simulink model "TST_EISGov_TrqLosEst"  (R2016b)
settings: Solver=FixedStepDiscrete  StartTime=0.0  StopTime=0.02  FixedStep=sampleTime  RelTol=1e-3
values from neighbouring files (symbols this model uses):
  testCase = 1    [initTST_EISGov_TrqLosEst_001.m]    (also in initTST_EISGov_TrqLosEst_002.m = 2; initTST_EISGov_TrqLosEst_003.m = 3; initTST_EISGov_TrqLosEst_004.m = 4)
libraries: simulink x9, UnitTest_Lib x4
settings Model: Creator=zhengjinyan  LastModifiedBy=zhengjinyan
settings DebuggingCC: SignalRangeChecking=error

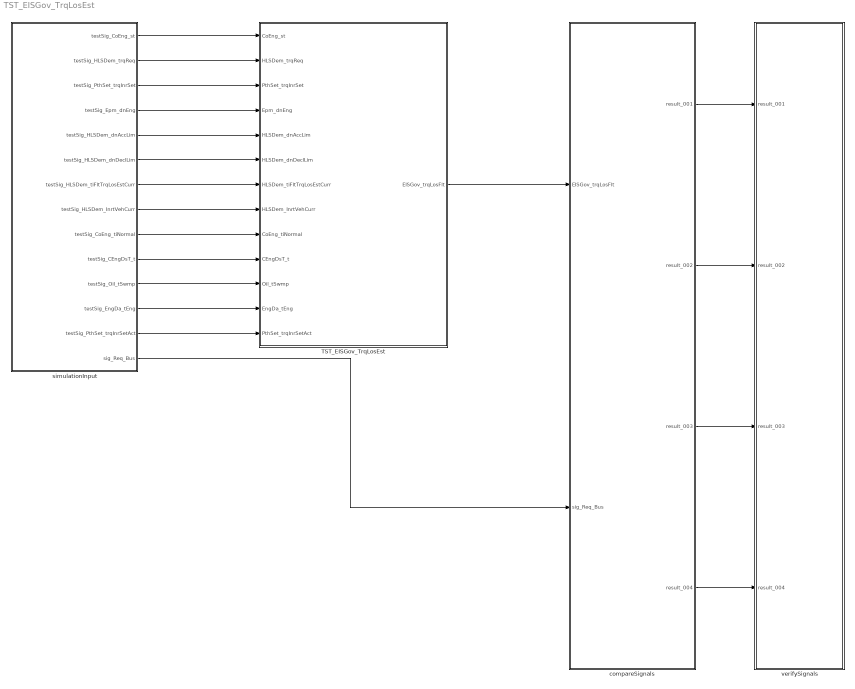
== system TST_EISGov_TrqLosEst ==
  TST_EISGov_TrqLosEst : Subsystem
  compareSignals : Subsystem
  simulationInput : Subsystem
  verifySignals : Subsystem
  wires:
  simulationInput/1(testSig_CoEng_st) -> TST_EISGov_TrqLosEst/1(CoEng_st)
  simulationInput/2(testSig_HLSDem_trqReq) -> TST_EISGov_TrqLosEst/2(HLSDem_trqReq)
  simulationInput/3(testSig_PthSet_trqInrSet) -> TST_EISGov_TrqLosEst/3(PthSet_trqInrSet)
  simulationInput/4(testSig_Epm_dnEng) -> TST_EISGov_TrqLosEst/4(Epm_dnEng)
  simulationInput/5(testSig_HLSDem_dnAccLim) -> TST_EISGov_TrqLosEst/5(HLSDem_dnAccLim)
  simulationInput/6(testSig_HLSDem_dnDeclLim) -> TST_EISGov_TrqLosEst/6(HLSDem_dnDeclLim)
  simulationInput/7(testSig_HLSDem_tiFltTrqLosEstCurr) -> TST_EISGov_TrqLosEst/7(HLSDem_tiFltTrqLosEstCurr)
  simulationInput/8(testSig_HLSDem_InrtVehCurr) -> TST_EISGov_TrqLosEst/8(HLSDem_InrtVehCurr)
  simulationInput/9(testSig_CoEng_tiNormal) -> TST_EISGov_TrqLosEst/9(CoEng_tiNormal)
  simulationInput/10(testSig_CEngDsT_t) -> TST_EISGov_TrqLosEst/10(CEngDsT_t)
  simulationInput/11(testSig_Oil_tSwmp) -> TST_EISGov_TrqLosEst/11(Oil_tSwmp)
  simulationInput/12(testSig_EngDa_tEng) -> TST_EISGov_TrqLosEst/12(EngDa_tEng)
  simulationInput/13(testSig_PthSet_trqInrSetAct) -> TST_EISGov_TrqLosEst/13(PthSet_trqInrSetAct)
  TST_EISGov_TrqLosEst/1(EISGov_trqLosFlt) -> compareSignals/1(EISGov_trqLosFlt)
  simulationInput/14(sig_Req_Bus) -> compareSignals/2(sig_Req_Bus)
  compareSignals/1(result_001) -> verifySignals/1(result_001)
  compareSignals/2(result_002) -> verifySignals/2(result_002)
  compareSignals/3(result_003) -> verifySignals/3(result_003)
  compareSignals/4(result_004) -> verifySignals/4(result_004)

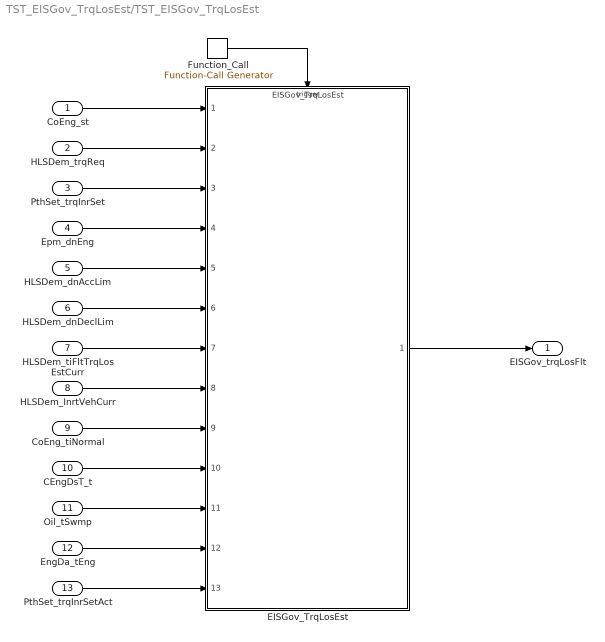
== system TST_EISGov_TrqLosEst/TST_EISGov_TrqLosEst ==
  CoEng_st : Inport
  HLSDem_trqReq : Inport  Port=2
  PthSet_trqInrSet : Inport  Port=3
  Epm_dnEng : Inport  Port=4
  HLSDem_dnAccLim : Inport  Port=5
  HLSDem_dnDeclLim : Inport  Port=6
  HLSDem_tiFltTrqLosEstCurr : Inport  Port=7
  HLSDem_InrtVehCurr : Inport  Port=8
  CoEng_tiNormal : Inport  Port=9
  CEngDsT_t : Inport  Port=10
  Oil_tSwmp : Inport  Port=11
  EngDa_tEng : Inport  Port=12
  PthSet_trqInrSetAct : Inport  Port=13
  EISGov_TrqLosEst : ModelReference  ModelNameDialog=EISGov_TrqLosEst  SimulationMode=Normal  ModelReferenceVersion=1.93  TriggerPortName=function  TriggerPortTriggerType=function-call  TriggerPortStatesWhenEnabling=held
  Function_Call : simulink/Ports & Subsystems/Function-Call Generator  sample_time=sampleTime  numberOfIterations=1
  EISGov_trqLosFlt : Outport
  wires:
  Function_Call/1 -> EISGov_TrqLosEst/Trigger
  CoEng_st/1 -> EISGov_TrqLosEst/1
  HLSDem_trqReq/1 -> EISGov_TrqLosEst/2
  PthSet_trqInrSet/1 -> EISGov_TrqLosEst/3
  Epm_dnEng/1 -> EISGov_TrqLosEst/4
  HLSDem_dnAccLim/1 -> EISGov_TrqLosEst/5
  HLSDem_dnDeclLim/1 -> EISGov_TrqLosEst/6
  HLSDem_tiFltTrqLosEstCurr/1 -> EISGov_TrqLosEst/7
  HLSDem_InrtVehCurr/1 -> EISGov_TrqLosEst/8
  CoEng_tiNormal/1 -> EISGov_TrqLosEst/9
  CEngDsT_t/1 -> EISGov_TrqLosEst/10
  Oil_tSwmp/1 -> EISGov_TrqLosEst/11
  EngDa_tEng/1 -> EISGov_TrqLosEst/12
  PthSet_trqInrSetAct/1 -> EISGov_TrqLosEst/13
  EISGov_TrqLosEst/1 -> EISGov_trqLosFlt/1

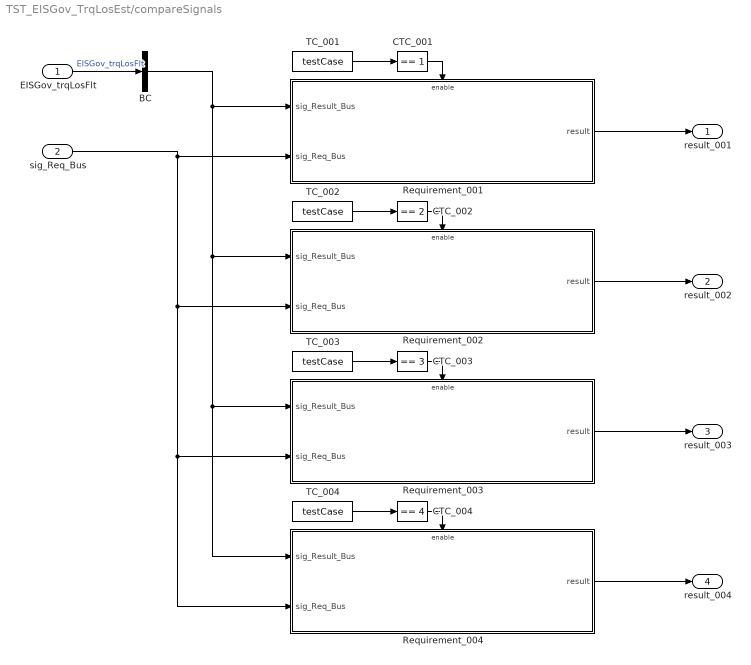
== system TST_EISGov_TrqLosEst/compareSignals ==
  EISGov_trqLosFlt : Inport
  sig_Req_Bus : Inport  Port=2
  BC : BusCreator  Inputs=1
  CTC_001 : simulink/Logic and Bit Operations/Compare To Constant  relop===  const=1  OutDataTypeStr=boolean
  CTC_002 : simulink/Logic and Bit Operations/Compare To Constant  relop===  const=2  OutDataTypeStr=boolean
  CTC_003 : simulink/Logic and Bit Operations/Compare To Constant  relop===  const=3  OutDataTypeStr=boolean
  CTC_004 : simulink/Logic and Bit Operations/Compare To Constant  relop===  const=4  OutDataTypeStr=boolean
  Requirement_001 : Subsystem
  Requirement_002 : Subsystem
  Requirement_003 : Subsystem
  Requirement_004 : Subsystem
  TC_001 : Constant  Value=testCase
  TC_002 : Constant  Value=testCase
  TC_003 : Constant  Value=testCase
  TC_004 : Constant  Value=testCase
  result_001 : Outport
  result_002 : Outport  Port=2
  result_003 : Outport  Port=3
  result_004 : Outport  Port=4
  wires:
  EISGov_trqLosFlt/1 -> BC/1  "EISGov_trqLosFlt"
  TC_001/1 -> CTC_001/1
  CTC_001/1 -> Requirement_001/Enable
  sig_Req_Bus/1 -> Requirement_003/2(sig_Req_Bus), Requirement_004/2(sig_Req_Bus), Requirement_002/2(sig_Req_Bus), Requirement_001/2(sig_Req_Bus)
  BC/1 -> Requirement_003/1(sig_Result_Bus), Requirement_004/1(sig_Result_Bus), Requirement_002/1(sig_Result_Bus), Requirement_001/1(sig_Result_Bus)
  Requirement_001/1(result) -> result_001/1
  TC_002/1 -> CTC_002/1
  CTC_002/1 -> Requirement_002/Enable
  Requirement_002/1(result) -> result_002/1
  TC_003/1 -> CTC_003/1
  CTC_003/1 -> Requirement_003/Enable
  Requirement_003/1(result) -> result_003/1
  TC_004/1 -> CTC_004/1
  CTC_004/1 -> Requirement_004/Enable
  Requirement_004/1(result) -> result_004/1

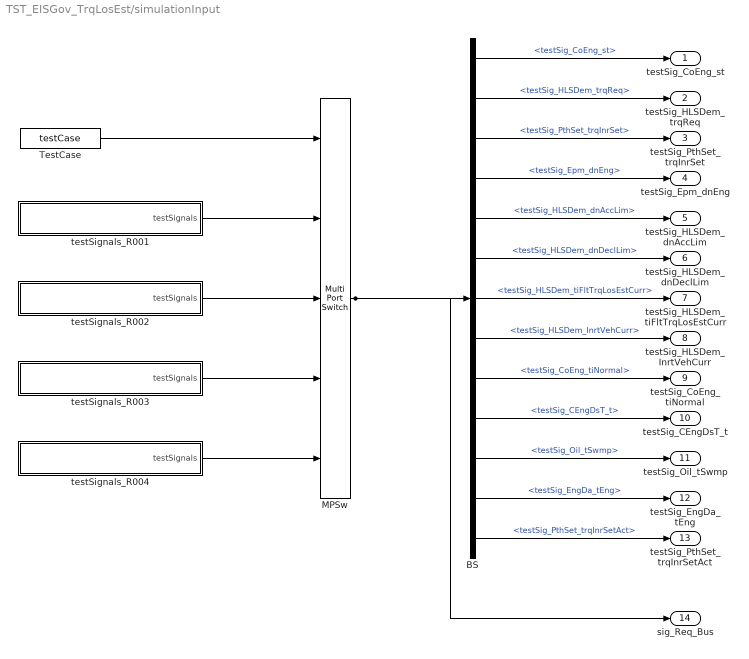
== system TST_EISGov_TrqLosEst/simulationInput ==
  BS : BusSelector  OutputSignals=testSig_CoEng_st,testSig_HLSDem_trqReq,testSig_PthSet_trqInrSet,testSig_Epm_dnEng,testSig_HLSDem_dnAccLim,testSig_HLSDem_dnDeclLim,testSig_HLSDem_tiFltTrqLosEstCurr,testSig_HLSDem_InrtVehCurr,testSig_CoEng_tiNormal,testSig_CEngDsT_t,testSig_Oil_tSwmp,testSig_EngDa_tEng,testSig_PthSet_trqInrSetAct
  MPSw : MultiPortSwitch  Inputs=4  SaturateOnIntegerOverflow=on  InputSameDT=on
  TestCase : Constant  Value=testCase
  testSignals_R001 : Subsystem
  testSignals_R002 : Subsystem
  testSignals_R003 : Subsystem
  testSignals_R004 : Subsystem
  testSig_CoEng_st : Outport
  testSig_HLSDem_trqReq : Outport  Port=2
  testSig_PthSet_trqInrSet : Outport  Port=3
  testSig_Epm_dnEng : Outport  Port=4
  testSig_HLSDem_dnAccLim : Outport  Port=5
  testSig_HLSDem_dnDeclLim : Outport  Port=6
  testSig_HLSDem_tiFltTrqLosEstCurr : Outport  Port=7
  testSig_HLSDem_InrtVehCurr : Outport  Port=8
  testSig_CoEng_tiNormal : Outport  Port=9
  testSig_CEngDsT_t : Outport  Port=10
  testSig_Oil_tSwmp : Outport  Port=11
  testSig_EngDa_tEng : Outport  Port=12
  testSig_PthSet_trqInrSetAct : Outport  Port=13
  sig_Req_Bus : Outport  Port=14
  wires:
  BS/1 -> testSig_CoEng_st/1  "<testSig_CoEng_st>"
  BS/2 -> testSig_HLSDem_trqReq/1  "<testSig_HLSDem_trqReq>"
  BS/3 -> testSig_PthSet_trqInrSet/1  "<testSig_PthSet_trqInrSet>"
  BS/4 -> testSig_Epm_dnEng/1  "<testSig_Epm_dnEng>"
  BS/5 -> testSig_HLSDem_dnAccLim/1  "<testSig_HLSDem_dnAccLim>"
  BS/6 -> testSig_HLSDem_dnDeclLim/1  "<testSig_HLSDem_dnDeclLim>"
  BS/7 -> testSig_HLSDem_tiFltTrqLosEstCurr/1  "<testSig_HLSDem_tiFltTrqLosEstCurr>"
  BS/8 -> testSig_HLSDem_InrtVehCurr/1  "<testSig_HLSDem_InrtVehCurr>"
  BS/9 -> testSig_CoEng_tiNormal/1  "<testSig_CoEng_tiNormal>"
  BS/10 -> testSig_CEngDsT_t/1  "<testSig_CEngDsT_t>"
  BS/11 -> testSig_Oil_tSwmp/1  "<testSig_Oil_tSwmp>"
  BS/12 -> testSig_EngDa_tEng/1  "<testSig_EngDa_tEng>"
  BS/13 -> testSig_PthSet_trqInrSetAct/1  "<testSig_PthSet_trqInrSetAct>"
  MPSw/1 -> BS/1, sig_Req_Bus/1
  TestCase/1 -> MPSw/1
  testSignals_R001/1(testSignals) -> MPSw/2
  testSignals_R002/1(testSignals) -> MPSw/3
  testSignals_R003/1(testSignals) -> MPSw/4
  testSignals_R004/1(testSignals) -> MPSw/5

== system TST_EISGov_TrqLosEst/verifySignals ==
  result_001 : Inport
  result_002 : Inport  Port=2
  result_003 : Inport  Port=3
  result_004 : Inport  Port=4
  Assertion_001 : Assertion  Enabled=off
  Assertion_002 : Assertion
  Assertion_003 : Assertion  Enabled=off
  Assertion_004 : Assertion  Enabled=off
  wires:
  result_001/1 -> Assertion_001/1
  result_002/1 -> Assertion_002/1
  result_003/1 -> Assertion_003/1
  result_004/1 -> Assertion_004/1

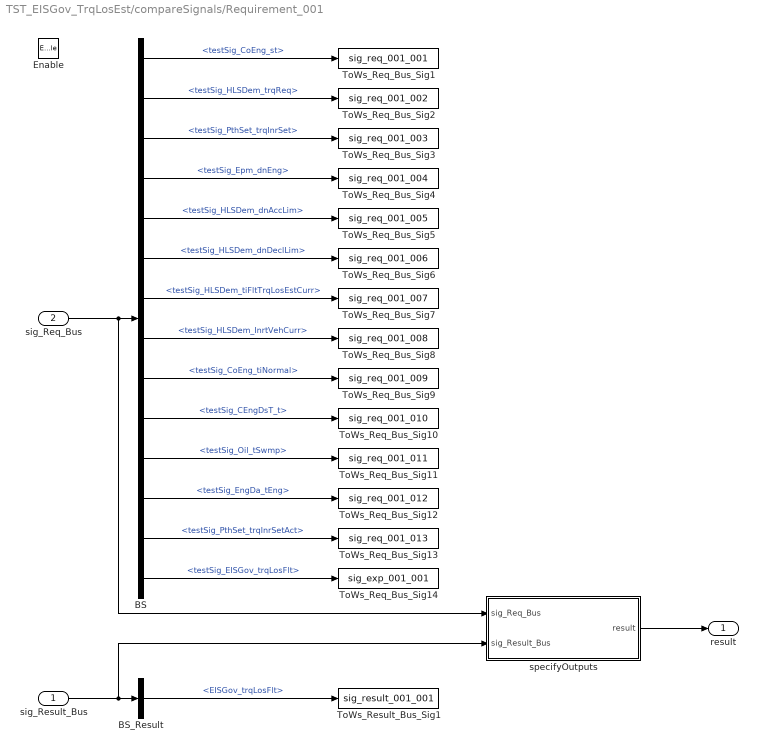
== system TST_EISGov_TrqLosEst/compareSignals/Requirement_001 ==
  sig_Result_Bus : Inport
  sig_Req_Bus : Inport  Port=2
  Enable : EnablePort
  BS : BusSelector  OutputSignals=testSig_CoEng_st,testSig_HLSDem_trqReq,testSig_PthSet_trqInrSet,testSig_Epm_dnEng,testSig_HLSDem_dnAccLim,testSig_HLSDem_dnDeclLim,testSig_HLSDem_tiFltTrqLosEstCurr,testSig_HLSDem_InrtVehCurr,testSig_CoEng_tiNormal,testSig_CEngDsT_t,testSig_Oil_tSwmp,testSig_EngDa_tEng,testSig_PthSet_trqInrSetAct,testSig_EISGov_trqLosFlt
  BS_Result : BusSelector  OutputSignals=EISGov_trqLosFlt
  ToWs_Req_Bus_Sig1 : ToWorkspace  VariableName=sig_req_001_001  SaveFormat=Structure With Time
  ToWs_Req_Bus_Sig10 : ToWorkspace  VariableName=sig_req_001_010  SaveFormat=Structure With Time
  ToWs_Req_Bus_Sig11 : ToWorkspace  VariableName=sig_req_001_011  SaveFormat=Structure With Time
  ToWs_Req_Bus_Sig12 : ToWorkspace  VariableName=sig_req_001_012  SaveFormat=Structure With Time
  ToWs_Req_Bus_Sig13 : ToWorkspace  VariableName=sig_req_001_013  SaveFormat=Structure With Time
  ToWs_Req_Bus_Sig14 : ToWorkspace  VariableName=sig_exp_001_001  SaveFormat=Structure With Time
  ToWs_Req_Bus_Sig2 : ToWorkspace  VariableName=sig_req_001_002  SaveFormat=Structure With Time
  ToWs_Req_Bus_Sig3 : ToWorkspace  VariableName=sig_req_001_003  SaveFormat=Structure With Time
  ToWs_Req_Bus_Sig4 : ToWorkspace  VariableName=sig_req_001_004  SaveFormat=Structure With Time
  ToWs_Req_Bus_Sig5 : ToWorkspace  VariableName=sig_req_001_005  SaveFormat=Structure With Time
  ToWs_Req_Bus_Sig6 : ToWorkspace  VariableName=sig_req_001_006  SaveFormat=Structure With Time
  ToWs_Req_Bus_Sig7 : ToWorkspace  VariableName=sig_req_001_007  SaveFormat=Structure With Time
  ToWs_Req_Bus_Sig8 : ToWorkspace  VariableName=sig_req_001_008  SaveFormat=Structure With Time
  ToWs_Req_Bus_Sig9 : ToWorkspace  VariableName=sig_req_001_009  SaveFormat=Structure With Time
  ToWs_Result_Bus_Sig1 : ToWorkspace  VariableName=sig_result_001_001  SaveFormat=Structure With Time
  specifyOutputs : Subsystem
  result : Outport
  wires:
  sig_Req_Bus/1 -> BS/1, specifyOutputs/1(sig_Req_Bus)
  BS/1 -> ToWs_Req_Bus_Sig1/1  "<testSig_CoEng_st>"
  BS/2 -> ToWs_Req_Bus_Sig2/1  "<testSig_HLSDem_trqReq>"
  BS/3 -> ToWs_Req_Bus_Sig3/1  "<testSig_PthSet_trqInrSet>"
  BS/4 -> ToWs_Req_Bus_Sig4/1  "<testSig_Epm_dnEng>"
  BS/5 -> ToWs_Req_Bus_Sig5/1  "<testSig_HLSDem_dnAccLim>"
  BS/6 -> ToWs_Req_Bus_Sig6/1  "<testSig_HLSDem_dnDeclLim>"
  BS/7 -> ToWs_Req_Bus_Sig7/1  "<testSig_HLSDem_tiFltTrqLosEstCurr>"
  BS/8 -> ToWs_Req_Bus_Sig8/1  "<testSig_HLSDem_InrtVehCurr>"
  BS/9 -> ToWs_Req_Bus_Sig9/1  "<testSig_CoEng_tiNormal>"
  BS/10 -> ToWs_Req_Bus_Sig10/1  "<testSig_CEngDsT_t>"
  BS/11 -> ToWs_Req_Bus_Sig11/1  "<testSig_Oil_tSwmp>"
  BS/12 -> ToWs_Req_Bus_Sig12/1  "<testSig_EngDa_tEng>"
  BS/13 -> ToWs_Req_Bus_Sig13/1  "<testSig_PthSet_trqInrSetAct>"
  BS/14 -> ToWs_Req_Bus_Sig14/1  "<testSig_EISGov_trqLosFlt>"
  sig_Result_Bus/1 -> BS_Result/1, specifyOutputs/2(sig_Result_Bus)
  BS_Result/1 -> ToWs_Result_Bus_Sig1/1  "<EISGov_trqLosFlt>"
  specifyOutputs/1(result) -> result/1

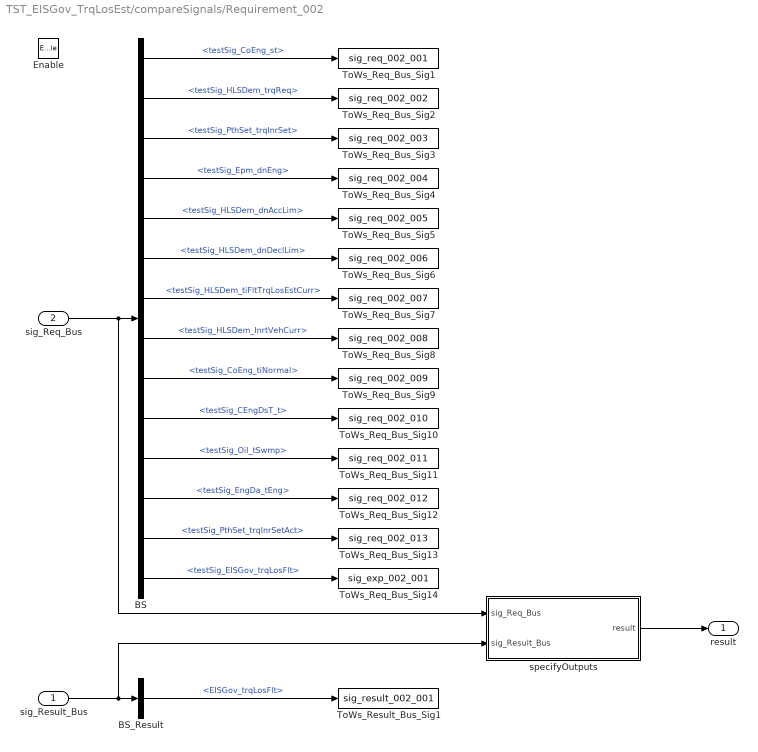
== system TST_EISGov_TrqLosEst/compareSignals/Requirement_002 ==
  sig_Result_Bus : Inport
  sig_Req_Bus : Inport  Port=2
  Enable : EnablePort
  BS : BusSelector  OutputSignals=testSig_CoEng_st,testSig_HLSDem_trqReq,testSig_PthSet_trqInrSet,testSig_Epm_dnEng,testSig_HLSDem_dnAccLim,testSig_HLSDem_dnDeclLim,testSig_HLSDem_tiFltTrqLosEstCurr,testSig_HLSDem_InrtVehCurr,testSig_CoEng_tiNormal,testSig_CEngDsT_t,testSig_Oil_tSwmp,testSig_EngDa_tEng,testSig_PthSet_trqInrSetAct,testSig_EISGov_trqLosFlt
  BS_Result : BusSelector  OutputSignals=EISGov_trqLosFlt
  ToWs_Req_Bus_Sig1 : ToWorkspace  VariableName=sig_req_002_001  SaveFormat=Structure With Time
  ToWs_Req_Bus_Sig10 : ToWorkspace  VariableName=sig_req_002_010  SaveFormat=Structure With Time
  ToWs_Req_Bus_Sig11 : ToWorkspace  VariableName=sig_req_002_011  SaveFormat=Structure With Time
  ToWs_Req_Bus_Sig12 : ToWorkspace  VariableName=sig_req_002_012  SaveFormat=Structure With Time
  ToWs_Req_Bus_Sig13 : ToWorkspace  VariableName=sig_req_002_013  SaveFormat=Structure With Time
  ToWs_Req_Bus_Sig14 : ToWorkspace  VariableName=sig_exp_002_001  SaveFormat=Structure With Time
  ToWs_Req_Bus_Sig2 : ToWorkspace  VariableName=sig_req_002_002  SaveFormat=Structure With Time
  ToWs_Req_Bus_Sig3 : ToWorkspace  VariableName=sig_req_002_003  SaveFormat=Structure With Time
  ToWs_Req_Bus_Sig4 : ToWorkspace  VariableName=sig_req_002_004  SaveFormat=Structure With Time
  ToWs_Req_Bus_Sig5 : ToWorkspace  VariableName=sig_req_002_005  SaveFormat=Structure With Time
  ToWs_Req_Bus_Sig6 : ToWorkspace  VariableName=sig_req_002_006  SaveFormat=Structure With Time
  ToWs_Req_Bus_Sig7 : ToWorkspace  VariableName=sig_req_002_007  SaveFormat=Structure With Time
  ToWs_Req_Bus_Sig8 : ToWorkspace  VariableName=sig_req_002_008  SaveFormat=Structure With Time
  ToWs_Req_Bus_Sig9 : ToWorkspace  VariableName=sig_req_002_009  SaveFormat=Structure With Time
  ToWs_Result_Bus_Sig1 : ToWorkspace  VariableName=sig_result_002_001  SaveFormat=Structure With Time
  specifyOutputs : Subsystem
  result : Outport
  wires:
  sig_Req_Bus/1 -> BS/1, specifyOutputs/1(sig_Req_Bus)
  BS/1 -> ToWs_Req_Bus_Sig1/1  "<testSig_CoEng_st>"
  BS/2 -> ToWs_Req_Bus_Sig2/1  "<testSig_HLSDem_trqReq>"
  BS/3 -> ToWs_Req_Bus_Sig3/1  "<testSig_PthSet_trqInrSet>"
  BS/4 -> ToWs_Req_Bus_Sig4/1  "<testSig_Epm_dnEng>"
  BS/5 -> ToWs_Req_Bus_Sig5/1  "<testSig_HLSDem_dnAccLim>"
  BS/6 -> ToWs_Req_Bus_Sig6/1  "<testSig_HLSDem_dnDeclLim>"
  BS/7 -> ToWs_Req_Bus_Sig7/1  "<testSig_HLSDem_tiFltTrqLosEstCurr>"
  BS/8 -> ToWs_Req_Bus_Sig8/1  "<testSig_HLSDem_InrtVehCurr>"
  BS/9 -> ToWs_Req_Bus_Sig9/1  "<testSig_CoEng_tiNormal>"
  BS/10 -> ToWs_Req_Bus_Sig10/1  "<testSig_CEngDsT_t>"
  BS/11 -> ToWs_Req_Bus_Sig11/1  "<testSig_Oil_tSwmp>"
  BS/12 -> ToWs_Req_Bus_Sig12/1  "<testSig_EngDa_tEng>"
  BS/13 -> ToWs_Req_Bus_Sig13/1  "<testSig_PthSet_trqInrSetAct>"
  BS/14 -> ToWs_Req_Bus_Sig14/1  "<testSig_EISGov_trqLosFlt>"
  sig_Result_Bus/1 -> BS_Result/1, specifyOutputs/2(sig_Result_Bus)
  BS_Result/1 -> ToWs_Result_Bus_Sig1/1  "<EISGov_trqLosFlt>"
  specifyOutputs/1(result) -> result/1

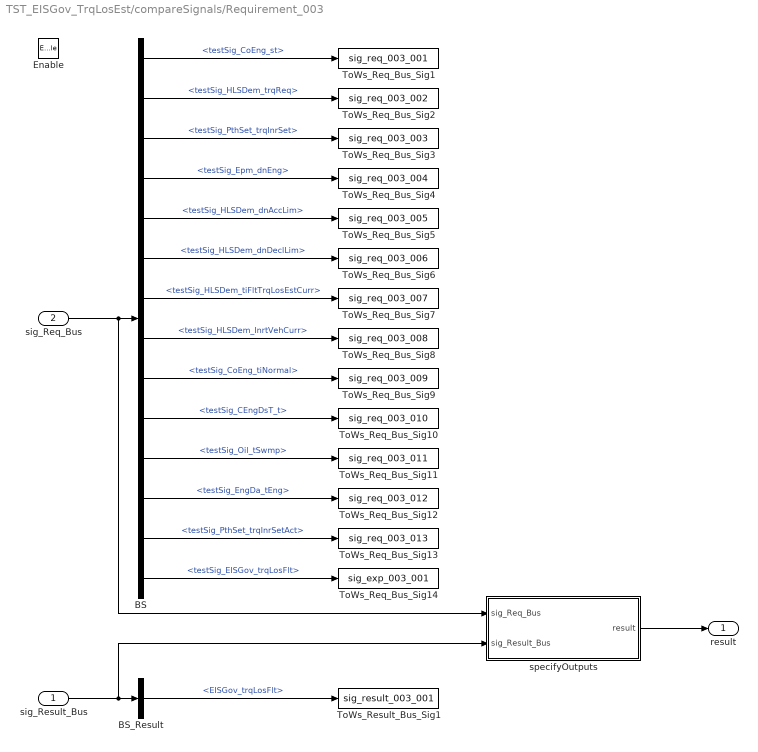
== system TST_EISGov_TrqLosEst/compareSignals/Requirement_003 ==
  sig_Result_Bus : Inport
  sig_Req_Bus : Inport  Port=2
  Enable : EnablePort
  BS : BusSelector  OutputSignals=testSig_CoEng_st,testSig_HLSDem_trqReq,testSig_PthSet_trqInrSet,testSig_Epm_dnEng,testSig_HLSDem_dnAccLim,testSig_HLSDem_dnDeclLim,testSig_HLSDem_tiFltTrqLosEstCurr,testSig_HLSDem_InrtVehCurr,testSig_CoEng_tiNormal,testSig_CEngDsT_t,testSig_Oil_tSwmp,testSig_EngDa_tEng,testSig_PthSet_trqInrSetAct,testSig_EISGov_trqLosFlt
  BS_Result : BusSelector  OutputSignals=EISGov_trqLosFlt
  ToWs_Req_Bus_Sig1 : ToWorkspace  VariableName=sig_req_003_001  SaveFormat=Structure With Time
  ToWs_Req_Bus_Sig10 : ToWorkspace  VariableName=sig_req_003_010  SaveFormat=Structure With Time
  ToWs_Req_Bus_Sig11 : ToWorkspace  VariableName=sig_req_003_011  SaveFormat=Structure With Time
  ToWs_Req_Bus_Sig12 : ToWorkspace  VariableName=sig_req_003_012  SaveFormat=Structure With Time
  ToWs_Req_Bus_Sig13 : ToWorkspace  VariableName=sig_req_003_013  SaveFormat=Structure With Time
  ToWs_Req_Bus_Sig14 : ToWorkspace  VariableName=sig_exp_003_001  SaveFormat=Structure With Time
  ToWs_Req_Bus_Sig2 : ToWorkspace  VariableName=sig_req_003_002  SaveFormat=Structure With Time
  ToWs_Req_Bus_Sig3 : ToWorkspace  VariableName=sig_req_003_003  SaveFormat=Structure With Time
  ToWs_Req_Bus_Sig4 : ToWorkspace  VariableName=sig_req_003_004  SaveFormat=Structure With Time
  ToWs_Req_Bus_Sig5 : ToWorkspace  VariableName=sig_req_003_005  SaveFormat=Structure With Time
  ToWs_Req_Bus_Sig6 : ToWorkspace  VariableName=sig_req_003_006  SaveFormat=Structure With Time
  ToWs_Req_Bus_Sig7 : ToWorkspace  VariableName=sig_req_003_007  SaveFormat=Structure With Time
  ToWs_Req_Bus_Sig8 : ToWorkspace  VariableName=sig_req_003_008  SaveFormat=Structure With Time
  ToWs_Req_Bus_Sig9 : ToWorkspace  VariableName=sig_req_003_009  SaveFormat=Structure With Time
  ToWs_Result_Bus_Sig1 : ToWorkspace  VariableName=sig_result_003_001  SaveFormat=Structure With Time
  specifyOutputs : Subsystem
  result : Outport
  wires:
  sig_Req_Bus/1 -> BS/1, specifyOutputs/1(sig_Req_Bus)
  BS/1 -> ToWs_Req_Bus_Sig1/1  "<testSig_CoEng_st>"
  BS/2 -> ToWs_Req_Bus_Sig2/1  "<testSig_HLSDem_trqReq>"
  BS/3 -> ToWs_Req_Bus_Sig3/1  "<testSig_PthSet_trqInrSet>"
  BS/4 -> ToWs_Req_Bus_Sig4/1  "<testSig_Epm_dnEng>"
  BS/5 -> ToWs_Req_Bus_Sig5/1  "<testSig_HLSDem_dnAccLim>"
  BS/6 -> ToWs_Req_Bus_Sig6/1  "<testSig_HLSDem_dnDeclLim>"
  BS/7 -> ToWs_Req_Bus_Sig7/1  "<testSig_HLSDem_tiFltTrqLosEstCurr>"
  BS/8 -> ToWs_Req_Bus_Sig8/1  "<testSig_HLSDem_InrtVehCurr>"
  BS/9 -> ToWs_Req_Bus_Sig9/1  "<testSig_CoEng_tiNormal>"
  BS/10 -> ToWs_Req_Bus_Sig10/1  "<testSig_CEngDsT_t>"
  BS/11 -> ToWs_Req_Bus_Sig11/1  "<testSig_Oil_tSwmp>"
  BS/12 -> ToWs_Req_Bus_Sig12/1  "<testSig_EngDa_tEng>"
  BS/13 -> ToWs_Req_Bus_Sig13/1  "<testSig_PthSet_trqInrSetAct>"
  BS/14 -> ToWs_Req_Bus_Sig14/1  "<testSig_EISGov_trqLosFlt>"
  sig_Result_Bus/1 -> BS_Result/1, specifyOutputs/2(sig_Result_Bus)
  BS_Result/1 -> ToWs_Result_Bus_Sig1/1  "<EISGov_trqLosFlt>"
  specifyOutputs/1(result) -> result/1

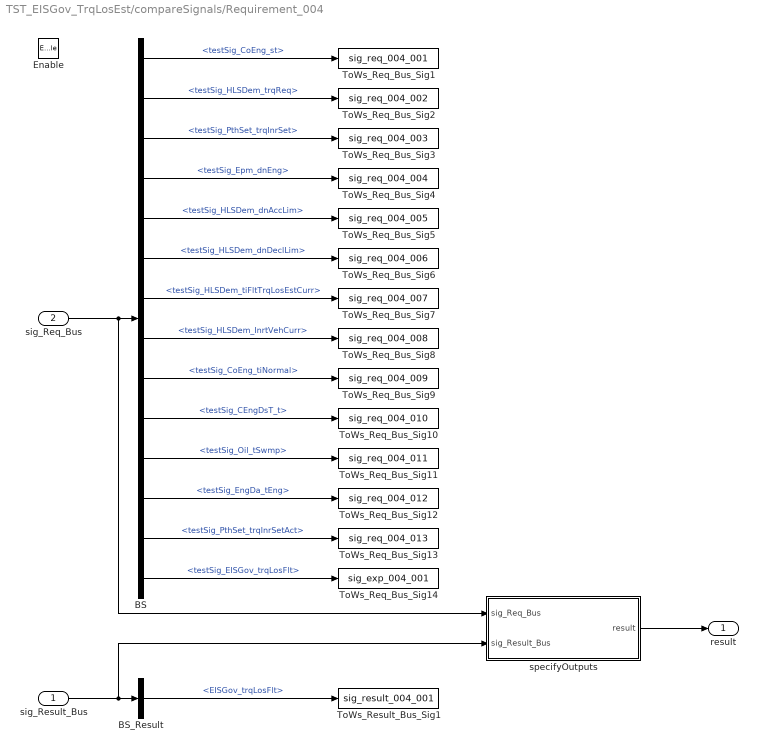
== system TST_EISGov_TrqLosEst/compareSignals/Requirement_004 ==
  sig_Result_Bus : Inport
  sig_Req_Bus : Inport  Port=2
  Enable : EnablePort
  BS : BusSelector  OutputSignals=testSig_CoEng_st,testSig_HLSDem_trqReq,testSig_PthSet_trqInrSet,testSig_Epm_dnEng,testSig_HLSDem_dnAccLim,testSig_HLSDem_dnDeclLim,testSig_HLSDem_tiFltTrqLosEstCurr,testSig_HLSDem_InrtVehCurr,testSig_CoEng_tiNormal,testSig_CEngDsT_t,testSig_Oil_tSwmp,testSig_EngDa_tEng,testSig_PthSet_trqInrSetAct,testSig_EISGov_trqLosFlt
  BS_Result : BusSelector  OutputSignals=EISGov_trqLosFlt
  ToWs_Req_Bus_Sig1 : ToWorkspace  VariableName=sig_req_004_001  SaveFormat=Structure With Time
  ToWs_Req_Bus_Sig10 : ToWorkspace  VariableName=sig_req_004_010  SaveFormat=Structure With Time
  ToWs_Req_Bus_Sig11 : ToWorkspace  VariableName=sig_req_004_011  SaveFormat=Structure With Time
  ToWs_Req_Bus_Sig12 : ToWorkspace  VariableName=sig_req_004_012  SaveFormat=Structure With Time
  ToWs_Req_Bus_Sig13 : ToWorkspace  VariableName=sig_req_004_013  SaveFormat=Structure With Time
  ToWs_Req_Bus_Sig14 : ToWorkspace  VariableName=sig_exp_004_001  SaveFormat=Structure With Time
  ToWs_Req_Bus_Sig2 : ToWorkspace  VariableName=sig_req_004_002  SaveFormat=Structure With Time
  ToWs_Req_Bus_Sig3 : ToWorkspace  VariableName=sig_req_004_003  SaveFormat=Structure With Time
  ToWs_Req_Bus_Sig4 : ToWorkspace  VariableName=sig_req_004_004  SaveFormat=Structure With Time
  ToWs_Req_Bus_Sig5 : ToWorkspace  VariableName=sig_req_004_005  SaveFormat=Structure With Time
  ToWs_Req_Bus_Sig6 : ToWorkspace  VariableName=sig_req_004_006  SaveFormat=Structure With Time
  ToWs_Req_Bus_Sig7 : ToWorkspace  VariableName=sig_req_004_007  SaveFormat=Structure With Time
  ToWs_Req_Bus_Sig8 : ToWorkspace  VariableName=sig_req_004_008  SaveFormat=Structure With Time
  ToWs_Req_Bus_Sig9 : ToWorkspace  VariableName=sig_req_004_009  SaveFormat=Structure With Time
  ToWs_Result_Bus_Sig1 : ToWorkspace  VariableName=sig_result_004_001  SaveFormat=Structure With Time
  specifyOutputs : Subsystem
  result : Outport
  wires:
  sig_Req_Bus/1 -> BS/1, specifyOutputs/1(sig_Req_Bus)
  BS/1 -> ToWs_Req_Bus_Sig1/1  "<testSig_CoEng_st>"
  BS/2 -> ToWs_Req_Bus_Sig2/1  "<testSig_HLSDem_trqReq>"
  BS/3 -> ToWs_Req_Bus_Sig3/1  "<testSig_PthSet_trqInrSet>"
  BS/4 -> ToWs_Req_Bus_Sig4/1  "<testSig_Epm_dnEng>"
  BS/5 -> ToWs_Req_Bus_Sig5/1  "<testSig_HLSDem_dnAccLim>"
  BS/6 -> ToWs_Req_Bus_Sig6/1  "<testSig_HLSDem_dnDeclLim>"
  BS/7 -> ToWs_Req_Bus_Sig7/1  "<testSig_HLSDem_tiFltTrqLosEstCurr>"
  BS/8 -> ToWs_Req_Bus_Sig8/1  "<testSig_HLSDem_InrtVehCurr>"
  BS/9 -> ToWs_Req_Bus_Sig9/1  "<testSig_CoEng_tiNormal>"
  BS/10 -> ToWs_Req_Bus_Sig10/1  "<testSig_CEngDsT_t>"
  BS/11 -> ToWs_Req_Bus_Sig11/1  "<testSig_Oil_tSwmp>"
  BS/12 -> ToWs_Req_Bus_Sig12/1  "<testSig_EngDa_tEng>"
  BS/13 -> ToWs_Req_Bus_Sig13/1  "<testSig_PthSet_trqInrSetAct>"
  BS/14 -> ToWs_Req_Bus_Sig14/1  "<testSig_EISGov_trqLosFlt>"
  sig_Result_Bus/1 -> BS_Result/1, specifyOutputs/2(sig_Result_Bus)
  BS_Result/1 -> ToWs_Result_Bus_Sig1/1  "<EISGov_trqLosFlt>"
  specifyOutputs/1(result) -> result/1

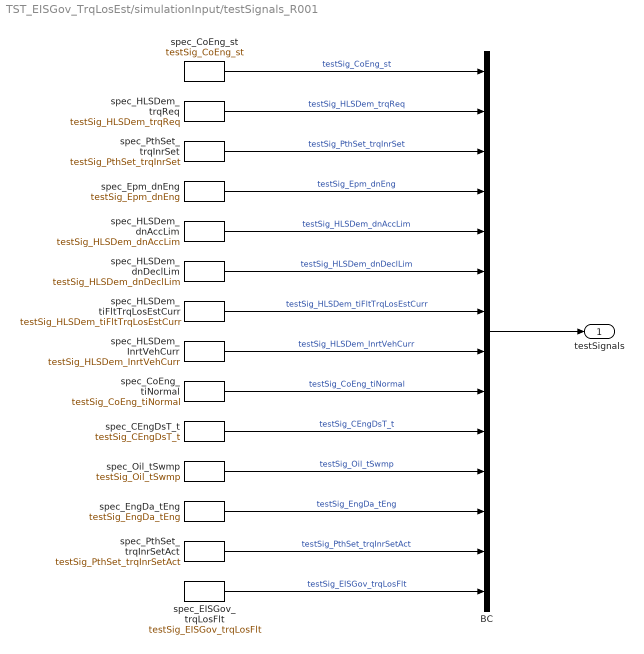
== system TST_EISGov_TrqLosEst/simulationInput/testSignals_R001 ==
  BC : BusCreator  Inputs=14
  spec_CEngDsT_t : FromWorkspace  VariableName=testSig_CEngDsT_t  Interpolate=off  OutputAfterFinalValue=Holding final value
  spec_CoEng_st : FromWorkspace  VariableName=testSig_CoEng_st  Interpolate=off  OutputAfterFinalValue=Holding final value
  spec_CoEng_tiNormal : FromWorkspace  VariableName=testSig_CoEng_tiNormal  Interpolate=off  OutputAfterFinalValue=Holding final value
  spec_EISGov_trqLosFlt : FromWorkspace  VariableName=testSig_EISGov_trqLosFlt  Interpolate=off  OutputAfterFinalValue=Holding final value
  spec_EngDa_tEng : FromWorkspace  VariableName=testSig_EngDa_tEng  Interpolate=off  OutputAfterFinalValue=Holding final value
  spec_Epm_dnEng : FromWorkspace  VariableName=testSig_Epm_dnEng  Interpolate=off  OutputAfterFinalValue=Holding final value
  spec_HLSDem_InrtVehCurr : FromWorkspace  VariableName=testSig_HLSDem_InrtVehCurr  Interpolate=off  OutputAfterFinalValue=Holding final value
  spec_HLSDem_dnAccLim : FromWorkspace  VariableName=testSig_HLSDem_dnAccLim  Interpolate=off  OutputAfterFinalValue=Holding final value
  spec_HLSDem_dnDeclLim : FromWorkspace  VariableName=testSig_HLSDem_dnDeclLim  Interpolate=off  OutputAfterFinalValue=Holding final value
  spec_HLSDem_tiFltTrqLosEstCurr : FromWorkspace  VariableName=testSig_HLSDem_tiFltTrqLosEstCurr  Interpolate=off  OutputAfterFinalValue=Holding final value
  spec_HLSDem_trqReq : FromWorkspace  VariableName=testSig_HLSDem_trqReq  Interpolate=off  OutputAfterFinalValue=Holding final value
  spec_Oil_tSwmp : FromWorkspace  VariableName=testSig_Oil_tSwmp  Interpolate=off  OutputAfterFinalValue=Holding final value
  spec_PthSet_trqInrSet : FromWorkspace  VariableName=testSig_PthSet_trqInrSet  Interpolate=off  OutputAfterFinalValue=Holding final value
  spec_PthSet_trqInrSetAct : FromWorkspace  VariableName=testSig_PthSet_trqInrSetAct  Interpolate=off  OutputAfterFinalValue=Holding final value
  testSignals : Outport
  wires:
  BC/1 -> testSignals/1
  spec_CoEng_st/1 -> BC/1  "testSig_CoEng_st"
  spec_HLSDem_trqReq/1 -> BC/2  "testSig_HLSDem_trqReq"
  spec_PthSet_trqInrSet/1 -> BC/3  "testSig_PthSet_trqInrSet"
  spec_Epm_dnEng/1 -> BC/4  "testSig_Epm_dnEng"
  spec_HLSDem_dnAccLim/1 -> BC/5  "testSig_HLSDem_dnAccLim"
  spec_HLSDem_dnDeclLim/1 -> BC/6  "testSig_HLSDem_dnDeclLim"
  spec_HLSDem_tiFltTrqLosEstCurr/1 -> BC/7  "testSig_HLSDem_tiFltTrqLosEstCurr"
  spec_HLSDem_InrtVehCurr/1 -> BC/8  "testSig_HLSDem_InrtVehCurr"
  spec_CoEng_tiNormal/1 -> BC/9  "testSig_CoEng_tiNormal"
  spec_CEngDsT_t/1 -> BC/10  "testSig_CEngDsT_t"
  spec_Oil_tSwmp/1 -> BC/11  "testSig_Oil_tSwmp"
  spec_EngDa_tEng/1 -> BC/12  "testSig_EngDa_tEng"
  spec_PthSet_trqInrSetAct/1 -> BC/13  "testSig_PthSet_trqInrSetAct"
  spec_EISGov_trqLosFlt/1 -> BC/14  "testSig_EISGov_trqLosFlt"

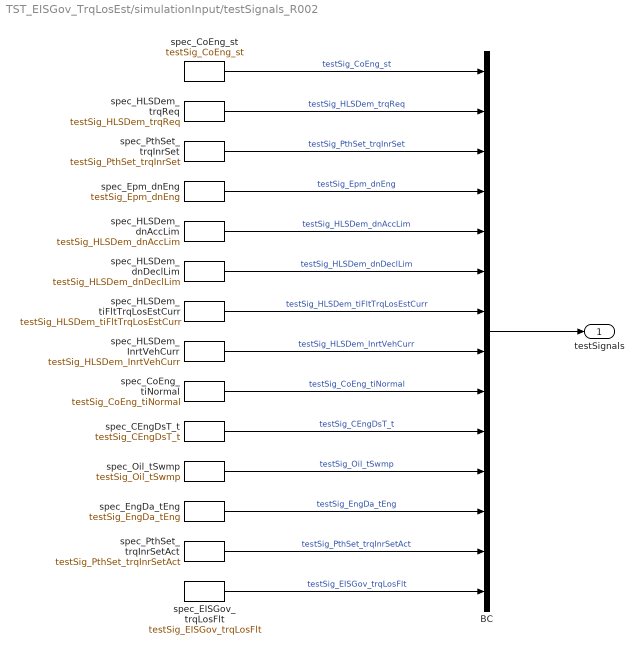
== system TST_EISGov_TrqLosEst/simulationInput/testSignals_R002 ==
  BC : BusCreator  Inputs=14
  spec_CEngDsT_t : FromWorkspace  VariableName=testSig_CEngDsT_t  Interpolate=off  OutputAfterFinalValue=Holding final value
  spec_CoEng_st : FromWorkspace  VariableName=testSig_CoEng_st  Interpolate=off  OutputAfterFinalValue=Holding final value
  spec_CoEng_tiNormal : FromWorkspace  VariableName=testSig_CoEng_tiNormal  Interpolate=off  OutputAfterFinalValue=Holding final value
  spec_EISGov_trqLosFlt : FromWorkspace  VariableName=testSig_EISGov_trqLosFlt  Interpolate=off  OutputAfterFinalValue=Holding final value
  spec_EngDa_tEng : FromWorkspace  VariableName=testSig_EngDa_tEng  Interpolate=off  OutputAfterFinalValue=Holding final value
  spec_Epm_dnEng : FromWorkspace  VariableName=testSig_Epm_dnEng  Interpolate=off  OutputAfterFinalValue=Holding final value
  spec_HLSDem_InrtVehCurr : FromWorkspace  VariableName=testSig_HLSDem_InrtVehCurr  Interpolate=off  OutputAfterFinalValue=Holding final value
  spec_HLSDem_dnAccLim : FromWorkspace  VariableName=testSig_HLSDem_dnAccLim  Interpolate=off  OutputAfterFinalValue=Holding final value
  spec_HLSDem_dnDeclLim : FromWorkspace  VariableName=testSig_HLSDem_dnDeclLim  Interpolate=off  OutputAfterFinalValue=Holding final value
  spec_HLSDem_tiFltTrqLosEstCurr : FromWorkspace  VariableName=testSig_HLSDem_tiFltTrqLosEstCurr  Interpolate=off  OutputAfterFinalValue=Holding final value
  spec_HLSDem_trqReq : FromWorkspace  VariableName=testSig_HLSDem_trqReq  Interpolate=off  OutputAfterFinalValue=Holding final value
  spec_Oil_tSwmp : FromWorkspace  VariableName=testSig_Oil_tSwmp  Interpolate=off  OutputAfterFinalValue=Holding final value
  spec_PthSet_trqInrSet : FromWorkspace  VariableName=testSig_PthSet_trqInrSet  Interpolate=off  OutputAfterFinalValue=Holding final value
  spec_PthSet_trqInrSetAct : FromWorkspace  VariableName=testSig_PthSet_trqInrSetAct  Interpolate=off  OutputAfterFinalValue=Holding final value
  testSignals : Outport
  wires:
  BC/1 -> testSignals/1
  spec_CoEng_st/1 -> BC/1  "testSig_CoEng_st"
  spec_HLSDem_trqReq/1 -> BC/2  "testSig_HLSDem_trqReq"
  spec_PthSet_trqInrSet/1 -> BC/3  "testSig_PthSet_trqInrSet"
  spec_Epm_dnEng/1 -> BC/4  "testSig_Epm_dnEng"
  spec_HLSDem_dnAccLim/1 -> BC/5  "testSig_HLSDem_dnAccLim"
  spec_HLSDem_dnDeclLim/1 -> BC/6  "testSig_HLSDem_dnDeclLim"
  spec_HLSDem_tiFltTrqLosEstCurr/1 -> BC/7  "testSig_HLSDem_tiFltTrqLosEstCurr"
  spec_HLSDem_InrtVehCurr/1 -> BC/8  "testSig_HLSDem_InrtVehCurr"
  spec_CoEng_tiNormal/1 -> BC/9  "testSig_CoEng_tiNormal"
  spec_CEngDsT_t/1 -> BC/10  "testSig_CEngDsT_t"
  spec_Oil_tSwmp/1 -> BC/11  "testSig_Oil_tSwmp"
  spec_EngDa_tEng/1 -> BC/12  "testSig_EngDa_tEng"
  spec_PthSet_trqInrSetAct/1 -> BC/13  "testSig_PthSet_trqInrSetAct"
  spec_EISGov_trqLosFlt/1 -> BC/14  "testSig_EISGov_trqLosFlt"

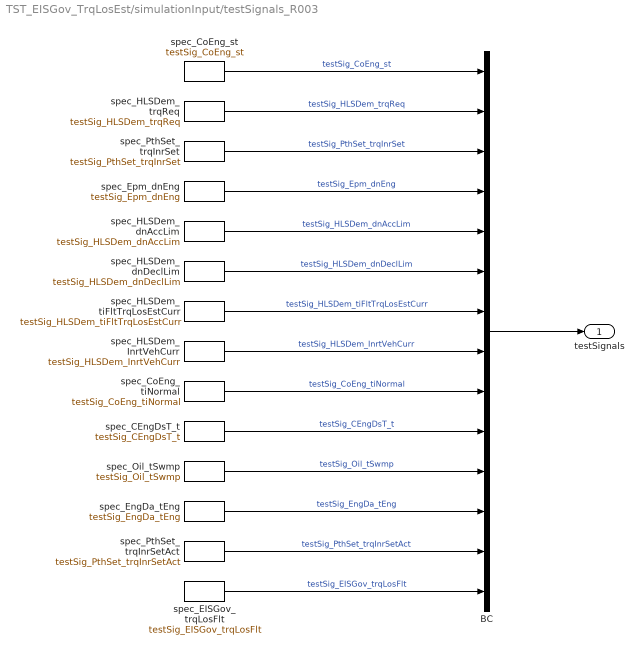
== system TST_EISGov_TrqLosEst/simulationInput/testSignals_R003 ==
  BC : BusCreator  Inputs=14
  spec_CEngDsT_t : FromWorkspace  VariableName=testSig_CEngDsT_t  Interpolate=off  OutputAfterFinalValue=Holding final value
  spec_CoEng_st : FromWorkspace  VariableName=testSig_CoEng_st  Interpolate=off  OutputAfterFinalValue=Holding final value
  spec_CoEng_tiNormal : FromWorkspace  VariableName=testSig_CoEng_tiNormal  Interpolate=off  OutputAfterFinalValue=Holding final value
  spec_EISGov_trqLosFlt : FromWorkspace  VariableName=testSig_EISGov_trqLosFlt  Interpolate=off  OutputAfterFinalValue=Holding final value
  spec_EngDa_tEng : FromWorkspace  VariableName=testSig_EngDa_tEng  Interpolate=off  OutputAfterFinalValue=Holding final value
  spec_Epm_dnEng : FromWorkspace  VariableName=testSig_Epm_dnEng  Interpolate=off  OutputAfterFinalValue=Holding final value
  spec_HLSDem_InrtVehCurr : FromWorkspace  VariableName=testSig_HLSDem_InrtVehCurr  Interpolate=off  OutputAfterFinalValue=Holding final value
  spec_HLSDem_dnAccLim : FromWorkspace  VariableName=testSig_HLSDem_dnAccLim  Interpolate=off  OutputAfterFinalValue=Holding final value
  spec_HLSDem_dnDeclLim : FromWorkspace  VariableName=testSig_HLSDem_dnDeclLim  Interpolate=off  OutputAfterFinalValue=Holding final value
  spec_HLSDem_tiFltTrqLosEstCurr : FromWorkspace  VariableName=testSig_HLSDem_tiFltTrqLosEstCurr  Interpolate=off  OutputAfterFinalValue=Holding final value
  spec_HLSDem_trqReq : FromWorkspace  VariableName=testSig_HLSDem_trqReq  Interpolate=off  OutputAfterFinalValue=Holding final value
  spec_Oil_tSwmp : FromWorkspace  VariableName=testSig_Oil_tSwmp  Interpolate=off  OutputAfterFinalValue=Holding final value
  spec_PthSet_trqInrSet : FromWorkspace  VariableName=testSig_PthSet_trqInrSet  Interpolate=off  OutputAfterFinalValue=Holding final value
  spec_PthSet_trqInrSetAct : FromWorkspace  VariableName=testSig_PthSet_trqInrSetAct  Interpolate=off  OutputAfterFinalValue=Holding final value
  testSignals : Outport
  wires:
  BC/1 -> testSignals/1
  spec_CoEng_st/1 -> BC/1  "testSig_CoEng_st"
  spec_HLSDem_trqReq/1 -> BC/2  "testSig_HLSDem_trqReq"
  spec_PthSet_trqInrSet/1 -> BC/3  "testSig_PthSet_trqInrSet"
  spec_Epm_dnEng/1 -> BC/4  "testSig_Epm_dnEng"
  spec_HLSDem_dnAccLim/1 -> BC/5  "testSig_HLSDem_dnAccLim"
  spec_HLSDem_dnDeclLim/1 -> BC/6  "testSig_HLSDem_dnDeclLim"
  spec_HLSDem_tiFltTrqLosEstCurr/1 -> BC/7  "testSig_HLSDem_tiFltTrqLosEstCurr"
  spec_HLSDem_InrtVehCurr/1 -> BC/8  "testSig_HLSDem_InrtVehCurr"
  spec_CoEng_tiNormal/1 -> BC/9  "testSig_CoEng_tiNormal"
  spec_CEngDsT_t/1 -> BC/10  "testSig_CEngDsT_t"
  spec_Oil_tSwmp/1 -> BC/11  "testSig_Oil_tSwmp"
  spec_EngDa_tEng/1 -> BC/12  "testSig_EngDa_tEng"
  spec_PthSet_trqInrSetAct/1 -> BC/13  "testSig_PthSet_trqInrSetAct"
  spec_EISGov_trqLosFlt/1 -> BC/14  "testSig_EISGov_trqLosFlt"

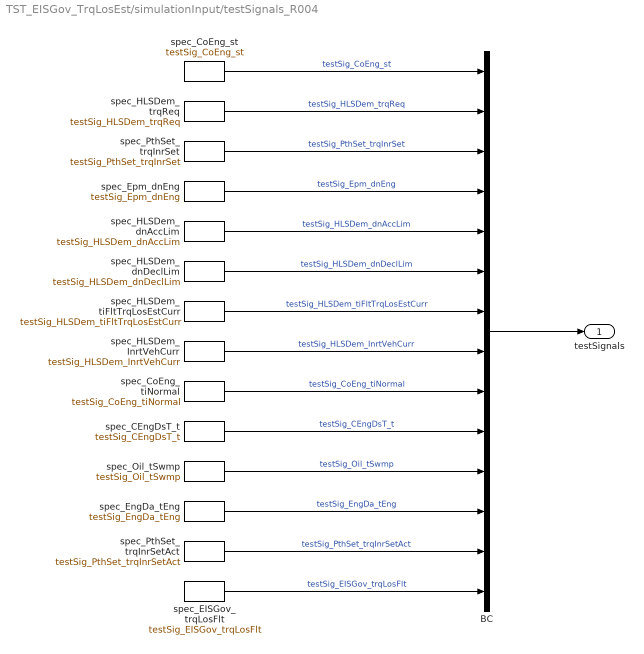
== system TST_EISGov_TrqLosEst/simulationInput/testSignals_R004 ==
  BC : BusCreator  Inputs=14
  spec_CEngDsT_t : FromWorkspace  VariableName=testSig_CEngDsT_t  Interpolate=off  OutputAfterFinalValue=Holding final value
  spec_CoEng_st : FromWorkspace  VariableName=testSig_CoEng_st  Interpolate=off  OutputAfterFinalValue=Holding final value
  spec_CoEng_tiNormal : FromWorkspace  VariableName=testSig_CoEng_tiNormal  Interpolate=off  OutputAfterFinalValue=Holding final value
  spec_EISGov_trqLosFlt : FromWorkspace  VariableName=testSig_EISGov_trqLosFlt  Interpolate=off  OutputAfterFinalValue=Holding final value
  spec_EngDa_tEng : FromWorkspace  VariableName=testSig_EngDa_tEng  Interpolate=off  OutputAfterFinalValue=Holding final value
  spec_Epm_dnEng : FromWorkspace  VariableName=testSig_Epm_dnEng  Interpolate=off  OutputAfterFinalValue=Holding final value
  spec_HLSDem_InrtVehCurr : FromWorkspace  VariableName=testSig_HLSDem_InrtVehCurr  Interpolate=off  OutputAfterFinalValue=Holding final value
  spec_HLSDem_dnAccLim : FromWorkspace  VariableName=testSig_HLSDem_dnAccLim  Interpolate=off  OutputAfterFinalValue=Holding final value
  spec_HLSDem_dnDeclLim : FromWorkspace  VariableName=testSig_HLSDem_dnDeclLim  Interpolate=off  OutputAfterFinalValue=Holding final value
  spec_HLSDem_tiFltTrqLosEstCurr : FromWorkspace  VariableName=testSig_HLSDem_tiFltTrqLosEstCurr  Interpolate=off  OutputAfterFinalValue=Holding final value
  spec_HLSDem_trqReq : FromWorkspace  VariableName=testSig_HLSDem_trqReq  Interpolate=off  OutputAfterFinalValue=Holding final value
  spec_Oil_tSwmp : FromWorkspace  VariableName=testSig_Oil_tSwmp  Interpolate=off  OutputAfterFinalValue=Holding final value
  spec_PthSet_trqInrSet : FromWorkspace  VariableName=testSig_PthSet_trqInrSet  Interpolate=off  OutputAfterFinalValue=Holding final value
  spec_PthSet_trqInrSetAct : FromWorkspace  VariableName=testSig_PthSet_trqInrSetAct  Interpolate=off  OutputAfterFinalValue=Holding final value
  testSignals : Outport
  wires:
  BC/1 -> testSignals/1
  spec_CoEng_st/1 -> BC/1  "testSig_CoEng_st"
  spec_HLSDem_trqReq/1 -> BC/2  "testSig_HLSDem_trqReq"
  spec_PthSet_trqInrSet/1 -> BC/3  "testSig_PthSet_trqInrSet"
  spec_Epm_dnEng/1 -> BC/4  "testSig_Epm_dnEng"
  spec_HLSDem_dnAccLim/1 -> BC/5  "testSig_HLSDem_dnAccLim"
  spec_HLSDem_dnDeclLim/1 -> BC/6  "testSig_HLSDem_dnDeclLim"
  spec_HLSDem_tiFltTrqLosEstCurr/1 -> BC/7  "testSig_HLSDem_tiFltTrqLosEstCurr"
  spec_HLSDem_InrtVehCurr/1 -> BC/8  "testSig_HLSDem_InrtVehCurr"
  spec_CoEng_tiNormal/1 -> BC/9  "testSig_CoEng_tiNormal"
  spec_CEngDsT_t/1 -> BC/10  "testSig_CEngDsT_t"
  spec_Oil_tSwmp/1 -> BC/11  "testSig_Oil_tSwmp"
  spec_EngDa_tEng/1 -> BC/12  "testSig_EngDa_tEng"
  spec_PthSet_trqInrSetAct/1 -> BC/13  "testSig_PthSet_trqInrSetAct"
  spec_EISGov_trqLosFlt/1 -> BC/14  "testSig_EISGov_trqLosFlt"

== system TST_EISGov_TrqLosEst/compareSignals/Requirement_001/specifyOutputs ==
  sig_Req_Bus : Inport
  sig_Result_Bus : Inport  Port=2
  AndN : Logic  Inputs=1
  BS_Req : BusSelector  OutputSignals=testSig_EISGov_trqLosFlt
  BS_Result : BusSelector  OutputSignals=EISGov_trqLosFlt
  Bitwise_And1 : simulink/Logic and Bit Operations/Bitwise Operator  logicop=AND  UseBitMask=off  BitMask=bin2dec('11011001')  BitMaskRealWorld=Stored Integer
  Scope : Scope
  Scope1 : Scope  NumInputPorts=2
  cmp_1 : UnitTest_Lib/RoughlyEqual  slope=2
  result_tws : ToWorkspace  VariableName=spec_result_001
  tws_1 : ToWorkspace  VariableName=spec_req_001_001
  result : Outport
  wires:
  sig_Req_Bus/1 -> BS_Req/1
  sig_Result_Bus/1 -> BS_Result/1
  AndN/1 -> result/1, result_tws/1
  BS_Req/1 -> cmp_1/1, Scope1/1  "<testSig_EISGov_trqLosFlt>"
  BS_Result/1 -> cmp_1/2, Scope1/2  "<EISGov_trqLosFlt>"
  cmp_1/1 -> Bitwise_And1/1
  Bitwise_And1/1 -> AndN/1, Scope/1, tws_1/1

== system TST_EISGov_TrqLosEst/compareSignals/Requirement_002/specifyOutputs ==
  sig_Req_Bus : Inport
  sig_Result_Bus : Inport  Port=2
  AndN : Logic  Inputs=1
  BS_Req : BusSelector  OutputSignals=testSig_EISGov_trqLosFlt
  BS_Result : BusSelector  OutputSignals=EISGov_trqLosFlt
  Bitwise_And1 : simulink/Logic and Bit Operations/Bitwise Operator  logicop=AND  UseBitMask=off  BitMask=bin2dec('11011001')  BitMaskRealWorld=Stored Integer
  Scope : Scope
  Scope1 : Scope  NumInputPorts=2
  cmp_1 : UnitTest_Lib/RoughlyEqual  slope=2
  result_tws : ToWorkspace  VariableName=spec_result_002
  tws_1 : ToWorkspace  VariableName=spec_req_002_001
  result : Outport
  wires:
  sig_Req_Bus/1 -> BS_Req/1
  sig_Result_Bus/1 -> BS_Result/1
  AndN/1 -> result/1, result_tws/1
  BS_Req/1 -> cmp_1/1, Scope1/1  "<testSig_EISGov_trqLosFlt>"
  BS_Result/1 -> cmp_1/2, Scope1/2  "<EISGov_trqLosFlt>"
  cmp_1/1 -> Bitwise_And1/1
  Bitwise_And1/1 -> AndN/1, Scope/1, tws_1/1

== system TST_EISGov_TrqLosEst/compareSignals/Requirement_003/specifyOutputs ==
  sig_Req_Bus : Inport
  sig_Result_Bus : Inport  Port=2
  AndN : Logic  Inputs=1
  BS_Req : BusSelector  OutputSignals=testSig_EISGov_trqLosFlt
  BS_Result : BusSelector  OutputSignals=EISGov_trqLosFlt
  Bitwise_And1 : simulink/Logic and Bit Operations/Bitwise Operator  logicop=AND  UseBitMask=off  BitMask=bin2dec('11011001')  BitMaskRealWorld=Stored Integer
  Scope : Scope
  Scope1 : Scope  NumInputPorts=2
  cmp_1 : UnitTest_Lib/RoughlyEqual  slope=2
  result_tws : ToWorkspace  VariableName=spec_result_003
  tws_1 : ToWorkspace  VariableName=spec_req_003_001
  result : Outport
  wires:
  sig_Req_Bus/1 -> BS_Req/1
  sig_Result_Bus/1 -> BS_Result/1
  AndN/1 -> result/1, result_tws/1
  BS_Req/1 -> cmp_1/1, Scope1/1  "<testSig_EISGov_trqLosFlt>"
  BS_Result/1 -> cmp_1/2, Scope1/2  "<EISGov_trqLosFlt>"
  cmp_1/1 -> Bitwise_And1/1
  Bitwise_And1/1 -> AndN/1, Scope/1, tws_1/1

== system TST_EISGov_TrqLosEst/compareSignals/Requirement_004/specifyOutputs ==
  sig_Req_Bus : Inport
  sig_Result_Bus : Inport  Port=2
  AndN : Logic  Inputs=1
  BS_Req : BusSelector  OutputSignals=testSig_EISGov_trqLosFlt
  BS_Result : BusSelector  OutputSignals=EISGov_trqLosFlt
  Bitwise_And1 : simulink/Logic and Bit Operations/Bitwise Operator  logicop=AND  UseBitMask=off  BitMask=bin2dec('11011001')  BitMaskRealWorld=Stored Integer
  Scope : Scope
  Scope1 : Scope  NumInputPorts=2
  cmp_1 : UnitTest_Lib/RoughlyEqual  slope=2
  result_tws : ToWorkspace  VariableName=spec_result_004
  tws_1 : ToWorkspace  VariableName=spec_req_004_001
  result : Outport
  wires:
  sig_Req_Bus/1 -> BS_Req/1
  sig_Result_Bus/1 -> BS_Result/1
  AndN/1 -> result/1, result_tws/1
  BS_Req/1 -> cmp_1/1, Scope1/1  "<testSig_EISGov_trqLosFlt>"
  BS_Result/1 -> cmp_1/2, Scope1/2  "<EISGov_trqLosFlt>"
  cmp_1/1 -> Bitwise_And1/1
  Bitwise_And1/1 -> AndN/1, Scope/1, tws_1/1
